simulink model "Versie2"  (R2019a)
(part 3 of 27)

  5 km series3/RConn1 -- Three-Phase Breaker 1/LConn1
  5 km series3/RConn2 -- Three-Phase Breaker 1/LConn2
  5 km series3/RConn3 -- Three-Phase Breaker 1/LConn3
  Three-Phase Breaker 2/RConn1 -- 5 km series3/LConn1
  Three-Phase Breaker 2/RConn2 -- 5 km series3/LConn2
  Three-Phase Breaker 2/RConn3 -- 5 km series3/LConn3
  Three-Phase Breaker 1/RConn1 -- BusC8/LConn1
  Three-Phase Breaker 1/RConn2 -- BusC8/LConn2
  Three-Phase Breaker 1/RConn3 -- BusC8/LConn3
  BusC12/RConn1 -- Three-Phase Breaker 2/LConn1
  BusC12/RConn2 -- Three-Phase Breaker 2/LConn2
  BusC12/RConn3 -- Three-Phase Breaker 2/LConn3
  Three-Phase Breaker 5/RConn3 -- 5 km series4/LConn3
  Three-Phase Breaker 5/RConn1 -- 5 km series4/LConn1
  5 km series4/RConn2 -- Three-Phase Breaker 3/LConn2
  5 km series4/RConn1 -- Three-Phase Breaker 3/LConn1
  BusC13/RConn1 -- Three-Phase Breaker 5/LConn1
  5 km series4/RConn3 -- Three-Phase Breaker 3/LConn3
  BusC13/RConn3 -- Three-Phase Breaker 5/LConn3
  BusC13/RConn2 -- Three-Phase Breaker 5/LConn2
  Three-Phase Breaker 5/RConn2 -- 5 km series4/LConn2
  Three-Phase Breaker 7/RConn3 -- 5 km series5/LConn3
  Three-Phase Breaker 7/RConn1 -- 5 km series5/LConn1
  5 km series5/RConn2 -- Three-Phase Breaker 6/LConn2
  5 km series5/RConn1 -- Three-Phase Breaker 6/LConn1
  BusC14/RConn1 -- Three-Phase Breaker 7/LConn1
  5 km series5/RConn3 -- Three-Phase Breaker 6/LConn3
  BusC14/RConn3 -- Three-Phase Breaker 7/LConn3
  BusC14/RConn2 -- Three-Phase Breaker 7/LConn2
  Three-Phase Breaker 7/RConn2 -- 5 km series5/LConn2
  Three-Phase Breaker 15/RConn3 -- 5 km series6/LConn3
  Three-Phase Breaker 15/RConn1 -- 5 km series6/LConn1
  5 km series6/RConn2 -- Three-Phase Breaker 8/LConn2
  5 km series6/RConn1 -- Three-Phase Breaker 8/LConn1
  BusC15/RConn1 -- Three-Phase Breaker 15/LConn1
  5 km series6/RConn3 -- Three-Phase Breaker 8/LConn3
  BusC15/RConn3 -- Three-Phase Breaker 15/LConn3
  BusC15/RConn2 -- Three-Phase Breaker 15/LConn2
  Three-Phase Breaker 15/RConn2 -- 5 km series6/LConn2
  BusC12/LConn1 -- BusC15/LConn1 -- BusC14/LConn1 -- BusC13/LConn1 -- BusC7/RConn1
  BusC12/LConn2 -- BusC15/LConn2 -- BusC14/LConn2 -- BusC13/LConn2 -- BusC7/RConn2
  BusC12/LConn3 -- BusC14/LConn3 -- BusC15/LConn3 -- BusC13/LConn3 -- BusC7/RConn3
  5 km series7/RConn2 -- Three-Phase Breaker 16/LConn2
  5 km series7/RConn1 -- Three-Phase Breaker 16/LConn1
  Three-Phase Breaker 17/RConn3 -- 5 km series7/LConn3
  BusC16/RConn3 -- Three-Phase Breaker 17/LConn3
  BusC16/RConn1 -- Three-Phase Breaker 17/LConn1
  Three-Phase Breaker 17/RConn1 -- 5 km series7/LConn1
  5 km series7/RConn3 -- Three-Phase Breaker 16/LConn3
  BusC16/RConn2 -- Three-Phase Breaker 17/LConn2
  Three-Phase Breaker 17/RConn2 -- 5 km series7/LConn2
  5 km series8/RConn2 -- Three-Phase Breaker 18/LConn2
  5 km series8/RConn1 -- Three-Phase Breaker 18/LConn1
  Three-Phase Breaker 19/RConn3 -- 5 km series8/LConn3
  BusC17/RConn3 -- Three-Phase Breaker 19/LConn3
  BusC17/RConn1 -- Three-Phase Breaker 19/LConn1
  Three-Phase Breaker 19/RConn1 -- 5 km series8/LConn1
  5 km series8/RConn3 -- Three-Phase Breaker 18/LConn3
  BusC17/RConn2 -- Three-Phase Breaker 19/LConn2
  Three-Phase Breaker 19/RConn2 -- 5 km series8/LConn2
  Three-Phase Breaker 16/RConn1 -- Three-Phase Breaker 18/RConn1 -- BusC7/LConn1
  Three-Phase Breaker 16/RConn2 -- Three-Phase Breaker 18/RConn2 -- BusC7/LConn2
  Three-Phase Breaker 16/RConn3 -- Three-Phase Breaker 18/RConn3 -- BusC7/LConn3
  2500 MVA X0/X1=2/RConn1 -- BusC17/LConn1 -- BusC16/LConn1
  BusC16/LConn2 -- BusC17/LConn2 -- 2500 MVA X0/X1=2/RConn2
  BusC16/LConn3 -- BusC17/LConn3 -- 2500 MVA X0/X1=2/RConn3
